simulink model "PennyFab_Deterministic"  (R2015b)
settings: Solver=VariableStepDiscrete  SolverMode=SingleTasking  StartTime=0.0  StopTime=1000  RelTol=1e-3
PostLoadFcn:
  | set_param(gcs, 'Location', [0 0 1750.0, 550.0]);
InitFcn:
  | warning('off','all');
StopFcn:
  | warning('on','all');
libraries: simeventslib x3, simulink x1
Description:
  | % LICENSE:  3-clause "Revised" or "New" or "Modified" BSD License.
  | % Copyright (c) 2015, Georgia Institute of Technology.
  | % All rights reserved.
  | %
  | % Redistribution and use in source and binary forms, with or without
  | % modification, are permitted provided that the following conditions are met:
  | %     * Redistributions of source code must retain the above copyright
  | %       notice, this list of conditions and the following disclaimer.
  | %     * Redistributions in binary form must reproduce the above copyright
  | %       notice, this list of conditions and the following disclaimer in the
  | %       documentation and/or other materials provided with the distribution.
  | %     * Neither the name of the Georgia Institute of Technology nor the
  | %       names of its contributors may be used to endorse or promote products
  | %       derived from this software without specific prior written permission.
  | %
  | % THIS SOFTWARE IS PROVIDED BY THE COPYRIGHT HOLDERS AND CONTRIBUTORS "AS IS" AND
  | % ANY EXPRESS OR IMPLIED WARRANTIES, INCLUDING, BUT NOT LIMITED TO, THE IMPLIED
  | % WARRANTIES OF MERCHANTABILITY AND FITNESS FOR A PARTICULAR PURPOSE ARE
  | % DISCLAIMED. IN NO EVENT SHALL THE GEORGIA INSTITUTE OF TECHNOLOGY BE LIABLE FOR
  | % ANY DIRECT, INDIRECT, INCIDENTAL, SPECIAL, EXEMPLARY, OR CONSEQUENTIAL DAMAGES
  | % (INCLUDING, BUT NOT LIMITED TO, PROCUREMENT OF SUBSTITUTE GOODS OR SERVICES;
  | % LOSS OF USE, DATA, OR PROFITS; OR BUSINESS INTERRUPTION) HOWEVER CAUSED AND
  | % ON ANY THEORY OF LIABILITY, WHETHER IN CONTRACT, STRICT LIABILITY, OR TORT
  | % (INCLUDING NEGLIGENCE OR OTHERWISE) ARISING IN ANY WAY OUT OF THE USE OF THIS
  | % SOFTWARE, EVEN IF ADVISED OF THE POSSIBILITY OF SUCH DAMAGE.
settings Model: Creator=tsprock3  LastModifiedBy=tsprock3
settings DataIOCC: SaveFormat=Array
settings OptimizationCC: BlockReduction=off  BooleanDataType=off
settings DebuggingCC: SaveWithParameterizedLinksMsg=none  UnderspecifiedInitializationDetection=Classic  MergeDetectMultiDrivingBlocksExec=none  SignalResolutionControl=TryResolveAllWithWarning
settings HardwareCC: ProdBitPerPointer=32  ProdLargestAtomicFloat=None  ProdIntDivRoundTo=Undefined  ProdEndianess=Unspecified  ProdWordSize=32  ProdHWDeviceType=32-bit Generic  TargetUnknown=on
settings GRTTargetCC: GeneratePreprocessorConditionals=Disable all
settings ConfigComp: CovModelRefEnable=Off

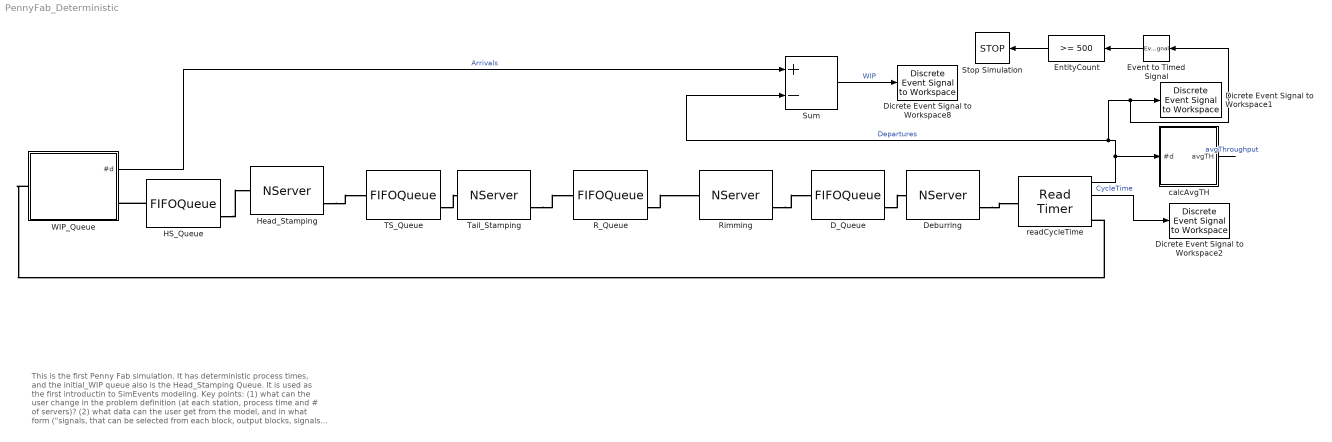
== system PennyFab_Deterministic ==
  note: This is the first Penny Fab simulation. It has deterministic process times, and the initial_WIP queue also is the Head_Stamping Queue.  It is used as the first introductin to SimEvents modeling. Key points: (1) what can the user change in the problem definition (at each station, process time and # of servers)? (2) what data can the user get from the model, and in what form ("signals, that can be selected from each block, output blocks, signals flagged for Simulation Data Explorer)?
      |
      | NB:  This model can be used to reproduce the results for both Penny Fab 1 and Penny Fab 2 in the textbook.
  D_Queue : FIFOQueue  StatNumberInBlock=on
      settings: OutputPortMap=o1
  Deburring : NServer  NumberOfServers=2  ServiceTime=3  StatNumberDeparted=on
  Dicrete Event Signal to Workspace1 : simeventslib/SimEvents Sinks/Discrete Event Signal to Workspace  VariableName=Departures  SaveFormat=Structure With Time  isMonitorOnly=off  isRecordIC=off
  Dicrete Event Signal to Workspace2 : simeventslib/SimEvents Sinks/Discrete Event Signal to Workspace  VariableName=CycleTime  SaveFormat=Structure With Time  isMonitorOnly=off  isRecordIC=off
  Dicrete Event Signal to Workspace8 : simeventslib/SimEvents Sinks/Discrete Event Signal to Workspace  VariableName=WIP  SaveFormat=Structure With Time  isMonitorOnly=off  isRecordIC=off
  EntityCount : simulink/Logic and Bit Operations/Compare To Constant  relop=>=  const=500  OutDataTypeStr=boolean
  Event to Timed Signal : EventToTimedSignal
  HS_Queue : FIFOQueue  StatNumberInBlock=on
      settings: OutputPortMap=o1
  Head_Stamping : NServer  NumberOfServers=1  ServiceTime=2  StatNumberDeparted=on
  R_Queue : FIFOQueue  StatNumberInBlock=on
      settings: OutputPortMap=o1
  Rimming : NServer  NumberOfServers=6  ServiceTime=10  StatNumberDeparted=on
  Stop Simulation : Stop
  Sum : Sum  Inputs=|+-
  TS_Queue : FIFOQueue  StatNumberInBlock=on
      settings: OutputPortMap=o1
  Tail_Stamping : NServer  NumberOfServers=2  ServiceTime=5  StatNumberDeparted=on
  WIP_Queue : Subsystem  mask{NumberOfEventsPerPeriod=4}
      mask prompts: NumberOfEventsPerPeriod "W := System WIP lLvel"
      mask TypeOptions NumberOfEventsPerPeriod: Generate/NumberOfEventsPerPeriod
      mask DialogControl DescTextVar Prompt: This parameter determines the total Work in Process (WIP) allowed in the closed system. The WIP level can impact the maximum throughput of the system.
  calcAvgTH : Subsystem
  readCycleTime : ReadTimer  TimerTag=CycleTime  StatNumberDeparted=on  StatTimeElapsed=on  StatAverageTimeElapsed=on
      settings: OutputPortMap=o0,o2,o3
  wires:
  readCycleTime/1 -> calcAvgTH/1(#d), Event to Timed Signal/1, Dicrete Event Signal to Workspace1/1, Sum/2  "Departures"
  Sum/1 -> Dicrete Event Signal to Workspace8/1  "WIP"
  WIP_Queue/1(#d) -> Sum/1  "Arrivals"
  readCycleTime/2 -> Dicrete Event Signal to Workspace2/1  "CycleTime"
  calcAvgTH/1(avgTH) -> ?  "avgThroughput"
  EntityCount/1 -> Stop Simulation/1
  Event to Timed Signal/1 -> EntityCount/1
  connections:
  Head_Stamping/RConn1 -- TS_Queue/LConn1
  Tail_Stamping/RConn1 -- R_Queue/LConn1
  Rimming/RConn1 -- D_Queue/LConn1
  Deburring/RConn1 -- readCycleTime/LConn1
  WIP_Queue/LConn1 -- readCycleTime/RConn1
  TS_Queue/RConn1 -- Tail_Stamping/LConn1
  R_Queue/RConn1 -- Rimming/LConn1
  D_Queue/RConn1 -- Deburring/LConn1
  HS_Queue/RConn1 -- Head_Stamping/LConn1
  HS_Queue/LConn1 -- WIP_Queue/RConn1

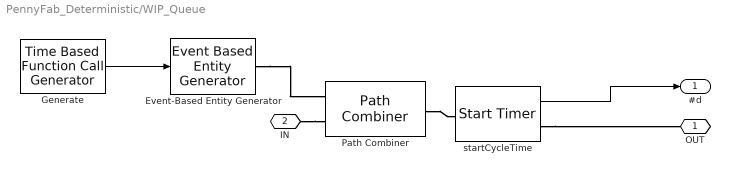
== system PennyFab_Deterministic/WIP_Queue ==
  Event-Based Entity Generator : EventBasedEntityGenerator  GenerateEntitiesUpon=Function call from port fcn
  Generate : TimeBasedFunctionCallGenerator  EventGenerationMode=Only at simulation start  NumberOfEventsPerPeriod=NumberOfEventsPerPeriod
  Path Combiner : PathCombiner  NumberInputPorts=2
  startCycleTime : StartTimer  TimerTag=CycleTime  TimerStartedOption=Restart  StatNumberDeparted=on
  OUT : PMIOPort  Port=1  Side=Right
  IN : PMIOPort  Port=2  Side=Left
  #d : Outport
  wires:
  Generate/1 -> Event-Based Entity Generator/1
  startCycleTime/1 -> #d/1
  connections:
  Path Combiner/RConn1 -- startCycleTime/LConn1
  startCycleTime/RConn1 -- OUT/RConn1
  IN/RConn1 -- Path Combiner/LConn2
  Event-Based Entity Generator/RConn1 -- Path Combiner/LConn1

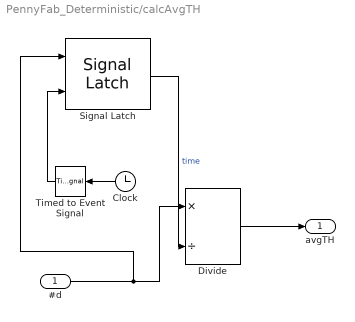
== system PennyFab_Deterministic/calcAvgTH ==
  #d : Inport
  Clock : Clock
  Divide : Product  Inputs=*/
  Signal Latch : SignalLatch  ReadMemoryUpon=Write to memory event
      settings: InputPortMap=u0,u2  OutputPortMap=o2
  Timed to Event Signal : TimedToEventSignal
  avgTH : Outport
  wires:
  #d/1 -> Signal Latch/1, Divide/1
  Timed to Event Signal/1 -> Signal Latch/2
  Signal Latch/1 -> Divide/2  "time"
  Clock/1 -> Timed to Event Signal/1
  Divide/1 -> avgTH/1
